simulink model "Lab1_3"  (R2024b)
settings: Solver=FixedStepAuto  StartTime=0.0  StopTime=inf  RelTol=1e-3  EnableMultiTasking=on
libraries: stm32f4xxblockslib x2
settings Model: STM32="{\"AnalogInput\":[{\"ID\":\"Basictest:1\"},{\"ID\":\"Basictest:24\"},{\"ID\":\"sosBasictest:52\"}],\"DigitalPortRead\":[{\"ID\":\"Basictest:37\"},{\"ID\":\"sosBasictest:58\"}]}"  Creator=newto  LastModifiedBy=newto
settings OptimizationCC: DefaultParameterBehavior=Inlined  EnhancedBackFolding=on  PassReuseOutputArgsAs=Individual arguments  ZeroExternalMemoryAtStartup=off  ZeroInternalMemoryAtStartup=off  MaxStackSize=512  OptimizeBlockOrder=speed  DifferentSizesBufferReuse=on  OptimizationCustomize=off  EfficientTunableParamExpr=on
settings DebuggingCC: ParameterTunabilityLossMsg=error
settings HardwareCC: ProdBitPerPointer=32  ProdBitPerSizeT=32  ProdBitPerPtrDiffT=32  ProdLargestAtomicInteger=Long  ProdLargestAtomicFloat=Double  ProdWordSize=32  ProdLongLongMode=on  ProdHWDeviceType=ARM Compatible->ARM Cortex-M
settings SFSimCC: MATLABDynamicMemAlloc=off
settings RTWCC: Description=Embedded Coder  SystemTargetFile=ert.tlc  HardwareBoard=STM32G4xx Based  TemplateMakefile=ert_default_tmf  Toolchain=GNU Tools for ARM Embedded Processors
settings CodeAppCC: ForceParamTrailComments=on  IgnoreCustomStorageClasses=off  OperatorAnnotations=on  SimulinkDataObjDesc=on  SFDataObjDesc=on  InsertBlockDesc=on
settings ERTTargetCC: TargetLangStandard=C99 (ISO)  CodeReplacementLibrary=ARM Cortex-M  ExtModeTransport=3  ExtModeStaticAlloc=on  ExtModeStaticAllocSize=2048  ExtModeMexFile=ext_xcp  ExtModeIntrfLevel=Level2 - Open

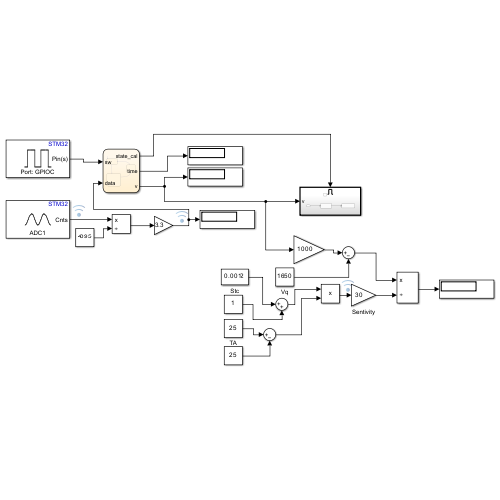
[thumbnail: Simulink's stored preview of the top-level diagram]
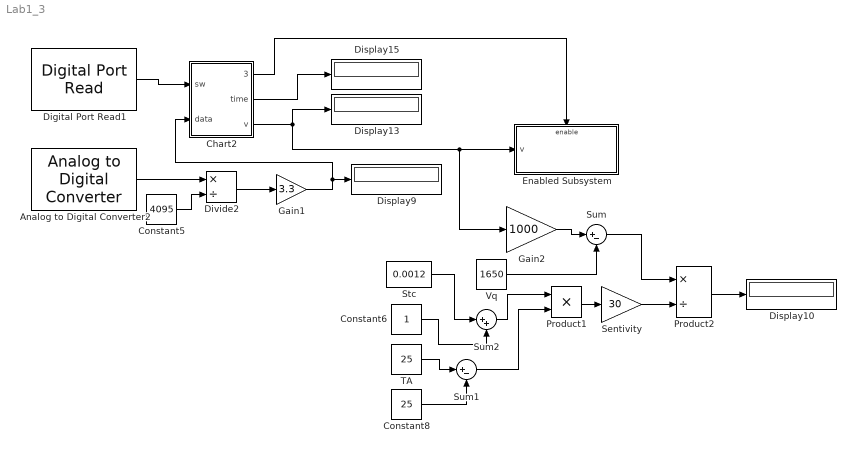
== system Lab1_3 ==
  Analog to Digital Converter2 : stm32f4xxblockslib/Analog to Digital Converter  ADCModule=ADC1  ConversionGroup=Regular  TriggerMode=Trigger and read  NumberOfConversions=1  EnableBufferConv=off  BufferLength=1  OutputStatus=off  SampleTime=-1  EnableSimPort=off  hoistedMaskSrc=ECSoC/ECSimCodegen/Analog to Digital Converter
  Chart2 : Stateflow chart  TreatAsAtomicUnit=on
      settings: PortSchema="{\"entries\":[{\"content\":{\"sides\":[{\"content\":{\"connectorIds\":[\"In1\",\"In2\"]},\"type\":\"ConnectorPlacement.EquallySpacedRectSide\",\"uuid\":\"5ec4fb54-4411-4273-b2fc-39c6053c04e2\"},{\"content\":{\"connectorIds\":[\"Out3\",\"Out1\",\"Out2\"],\"side\":\"RIGHT\"},\"type\":\"ConnectorPlacement.EquallySpacedRectSide\",\"uuid\":\"7d4fd8d5-e2fa-4e95-bf28-1a2de38ed455\"},{\"content\":{\"side\":\"TOP\"},\"type\":\"ConnectorPlacement.EquallySpacedRectSide\",\"uuid\":\"af9cccf0-b101-4036-9308-22282fced5b0\"}]},\"type\":\"ConnectorPlacement.EquallySpacedConnector\",\"uuid\":\"092a4951-e742-4edd-894e-38e3bc1df521\"}],\"packageUris\":[\"http://schema.mathworks.com/mf0/Connector/R2020b\"],\"version\":\"1.0\"}"
  Constant5 : Constant  Value=4095
  Constant6 : Constant
  Constant8 : Constant  Value=25
  Digital Port Read1 : stm32f4xxblockslib/Digital Port Read  PortName=GPIOC  PinNumber=13  ReadOperation=on  IOAsArray=on  SampleTime=-1  EnableSimPort=off  hoistedMaskSrc=ECSoC/ECSimCodegen/Digital Port Read
      settings: LibrarySourceBlock=stm32g4xxblockslib/Digital Port Read
  Display{9..10,13,15} (4 alike) : Display
  Divide2 : Product  Inputs=*/
  Enabled Subsystem : Subsystem  TreatAsAtomicUnit=on
  Gain1 : Gain  Gain=3.3
  Gain2 : Gain  Gain=1000
  Product1 : Product
  Product2 : Product  Inputs=*/
  Sentivity : Gain  Gain=30
  Stc : Constant  Value=0.0012
  Sum : Sum  Inputs=|+-
  Sum1 : Sum  Inputs=|+-
  Sum2 : Sum  Inputs=|++
  TA : Constant  Value=25
  Vq : Constant  Value=1650
  wires:
  Chart2/3(state_cal) -> Enabled Subsystem/Enable
  Chart2/2(v) -> Enabled Subsystem/1(v), Gain2/1, Display13/1
  Constant5/1 -> Divide2/2
  Divide2/1 -> Gain1/1
  Digital Port Read1/1 -> Chart2/1(sw)
  Analog to Digital Converter2/1 -> Divide2/1
  Chart2/1(time) -> Display15/1
  Gain1/1 -> Chart2/2(data), Display9/1
  Vq/1 -> Sum/2
  Gain2/1 -> Sum/1
  TA/1 -> Sum1/1
  Constant8/1 -> Sum1/2
  Stc/1 -> Sum2/1
  Constant6/1 -> Sum2/2
  Sum2/1 -> Product1/1
  Sum1/1 -> Product1/2
  Product1/1 -> Sentivity/1
  Sentivity/1 -> Product2/2
  Sum/1 -> Product2/1
  Product2/1 -> Display10/1

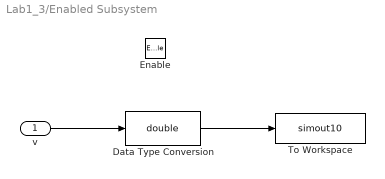
== system Lab1_3/Enabled Subsystem ==
  v : Inport
  Enable : EnablePort
  Data Type Conversion : DataTypeConversion  OutDataTypeStr=double  SaturateOnIntegerOverflow=off  RndMeth=Floor
  To Workspace : ToWorkspace  VariableName=simout10  SampleTime=-1
      settings: Save2DSignal=2-D array (concatenate along first dimension)
  wires:
  v/1 -> Data Type Conversion/1
  Data Type Conversion/1 -> To Workspace/1

== stateflow chart Lab1_3/Chart2 ==
  state initial
    v ;
    time = 0;
    state_cal = 0;
  state StopCount
    entry:
    state_cal = 1
  state CountData
    entry:
    v = data - data;
    during:
    v = v + data
    time=time+0.00714285714
    data
    exit:
    v = v/140;
  (default) -> initial
  StopCount -> initial
  initial -> CountData : [sw==1]
  CountData -> StopCount : [time>=1]
  data: sw input; data input; time output; v output; state_cal output
